simulink model "TRAMI_STEP_AT_vehicle_ver01_R2018b"  (R2018b)
settings: Solver=ode8  StartTime=0  StopTime=end_time  FixedStep=sampling_time  RelTol=1e-3
StartFcn:
  | csvwrite('simstart.csv',1)
StopFcn:
  | csvwrite('simstop.csv',1)
values from neighbouring files (symbols this model uses):
  sampling_time = 0.0025    [METI_TRAMI_Thermal_ver01_Jmaab_PreLoad.m]
undefined symbols (not defined in the file or in its folder): ACC_D_Gain, ACC_I_Gain, ACC_P_Gain, ALT_CNT_ALT_OFF_RPM_HYS_rpm, ALT_CNT_ALT_ON_RPM_HYS_rpm, ALT_CNT_Alter_V_BASE_V, ALT_CNT_Alter_V_Kaisei_V, ALT_CNT_flag_disable_kaisei, ALT_CNT_V_Battely_Kudo_V, ALT_PNT_ALT_GDCurrent_A, ALT_PNT_ALT_GDVolt_V, ALT_PNT_Alter_limit_Current_V_table, ALT_PNT_Alter_limit_Current_V_table_x_rpm, ALT_PNT_Alter_trq_Nm_map, ALT_PNT_Alter_trq_Nm_map_x_rpm, ALT_PNT_Alter_trq_Nm_map_y_Current_A, ALT_PNT_Alter_trq_Nm_map_z_Volt_tgt_V, ALT_PNT_eta_pulley_alt, ALT_PNT_Gain_Alt_v_del, ALT_PNT_ratio_pulley_alt, ALT_PNT_Tau_Alternator_V_tgt_s, ALT_PNT_trq_alter_output_LL_Nm, BK_PNT_Pow_UL, BK_PNT_Tau_brake, Brk_LL, Brk_PGain, Brk_UL, BT_PNT_Lo_Capa_lo_batt_F, BT_PNT_Lo_ocv_SOC_lo_batt_OCV_V_table, BT_PNT_Lo_ocv_SOC_lo_batt_OCV_V_table_x_SOC, BT_PNT_Lo_R_lo_batt_ohm, BT_PNT_Lo_SOC_MAX_lo_batt, BT_PNT_Lo_SOC_MIN_lo_batt, BT_PNT_Lo_SOC_START_lo_batt, BT_PNT_Lo_V_start_ocv, Driver_Brake_Const1, Driver_Brake_Const3, Driver_Brake_Switch_Const2, Driver_Brk_sh, drivmode_ACC, drivmode_CONST, drivmode_GensokuKaisei, drivmode_GensokuRikko, drivmode_STOP, EL_PNT_R_bodyelec_lo_ohm, ENG_CNT_Accel_LL, ENG_CNT_Accel_UL, ENG_CNT_brak_idlestop, ENG_CNT_flag_idle_stop_exe, ENG_CNT_gain_p_per_isc, ENG_CNT_IdleSpeed_Const, ENG_CNT_omg_eng_fuelcut_rpm, ENG_CNT_per_isc_max, ENG_CNT_per_isc_min, ENG_CNT_per_throttle_fuelcut, ENG_CNT_per_throttle_isc_fb, ENG_CNT_Starter_timer_Const_s, ENG_CNT_Throttle_LL, ENG_CNT_Throttle_UL, ENG_CNT_V_car_idlestop_kmph ... (+29)
libraries: METI_Lib_vehicle_model x18, simulink x4, AZAPA_Lib_vehicle_model x1
(part 1 of 2)
settings Model: SimulationMode=accelerator  Creator=nishimura  LastModifiedBy=kotaroy
settings SolverCC: AlgebraicLoopSolver=LineSearch
settings DataIOCC: SaveFormat=Array  SaveOutput=off  SignalLogging=off  DSMLogging=off  SaveTime=off
settings OptimizationCC: BlockReduction=off  BooleanDataType=off  EfficientMapNaN2IntZero=off  LifeSpan=inf
settings DebuggingCC: SaveWithParameterizedLinksMsg=none  UnderspecifiedInitializationDetection=Classic  MergeDetectMultiDrivingBlocksExec=none  SignalResolutionControl=TryResolveAllWithWarning  ParameterPrecisionLossMsg=none  AllowSymbolicDim=off  StrictBusMsg=ErrorOnBusTreatedAsVector  SFUnexpectedBacktrackingDiag=warning  SFNoUnconditionalDefaultTransitionDiag=warning  SFExecutionAtInitializationDiag=none
settings HardwareCC: ProdBitPerPointer=32  ProdBitPerSizeT=32  ProdBitPerPtrDiffT=32  ProdLargestAtomicFloat=None  ProdIntDivRoundTo=Undefined  ProdEndianess=Unspecified  ProdWordSize=32  ProdHWDeviceType=32-bit Generic  TargetBitPerPointer=64  TargetBitPerSizeT=64  TargetBitPerPtrDiffT=64  TargetLongLongMode=on  TargetIntDivRoundTo=Zero  TargetEndianess=LittleEndian  TargetWordSize=64  TargetHWDeviceType=MATLAB Host  ProdEqTarget=off
settings ModelReferenceCC: PropagateSignalLabelsOutOfModel=off
settings SFSimCC: SimUseLocalCustomCode=off
settings CodeAppCC: MaxIdLength=128
settings GRTTargetCC: TargetLangStandard=C89/C90 (ANSI)  CombineOutputUpdateFcns=off  GRTInterface=on
settings ConfigComp: CovMetricSettings=dw  CovHtmlReporting=on  CovSaveCumulativeToWorkspaceVar=on  CovSaveSingleToWorkspaceVar=on  CovExternalEMLEnable=off  CovSFcnEnable=off

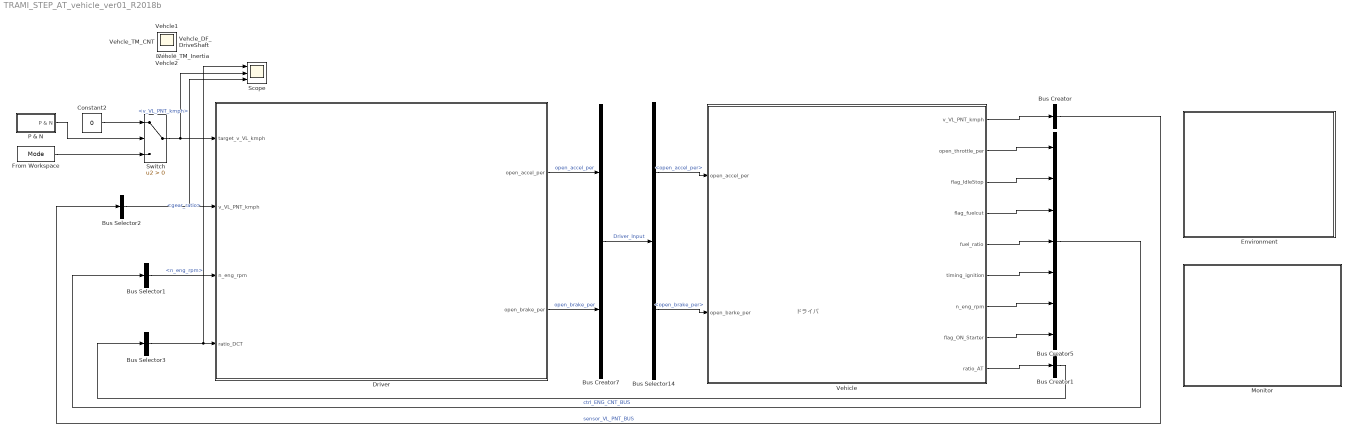
== system TRAMI_STEP_AT_vehicle_ver01_R2018b ==
  note: ドライバ
  Bus Creator : BusCreator  Inputs=1
  Bus Creator1 : BusCreator  Inputs=1
  Bus Creator5 : BusCreator  Inputs=7
  Bus Creator7 : BusCreator  Inputs=2
  Bus Selector1 : BusSelector  OutputSignals=n_eng_rpm
  Bus Selector14 : BusSelector  OutputSignals=open_accel_per,open_brake_per
  Bus Selector2 : BusSelector  OutputSignals=v_VL_PNT_kmph
  Bus Selector3 : BusSelector  OutputSignals=gear_ratio
  Constant2 : Constant  Value=0
  Driver : Subsystem
      mask Display: image(imread('picture\ドライバ.png'))
  Environment : Subsystem
      mask Display: image(imread('picture\外部環境.png'))
  From Workspace : FromWorkspace  VariableName=Mode  SampleTime=0  OutputAfterFinalValue=Holding final value
  Monitor : Subsystem
  P & N : Subsystem
  Scope : Scope  NumInputPorts=3
  Switch : Switch  Criteria=u2 > Threshold
  Vehicle : Subsystem
      mask Display: image(imread('picture\電気負荷.png'))
  Driver1 : Scope
  Vehcle1 : Scope
  Vehcle2 : Scope
  Vehcle_DF_DriveShaft : Scope
  Vehcle_TM_CNT : Scope
  Vehcle_TM_Inertia : Scope
  wires:
  Bus Creator7/1 -> Bus Selector14/1  "Driver_Input"
  Bus Creator/1 -> Bus Selector2/1  "sensor_VL_PNT_BUS"
  Bus Creator5/1 -> Bus Selector1/1  "ctrl_ENG_CNT_BUS"
  Vehicle/1(v_VL_PNT_kmph) -> Bus Creator/1
  Vehicle/2(open_throttle_per) -> Bus Creator5/1
  Vehicle/3(flag_IdleStop) -> Bus Creator5/2
  Vehicle/4(flag_fuelcut) -> Bus Creator5/3
  Vehicle/5(fuel_ratio) -> Bus Creator5/4
  Vehicle/6(timing_ignition) -> Bus Creator5/5
  Vehicle/7(n_eng_rpm) -> Bus Creator5/6
  Vehicle/8(flag_ON_Starter) -> Bus Creator5/7
  Bus Selector14/1 -> Vehicle/1(open_accel_per)  "<open_accel_per>"
  Bus Selector14/2 -> Vehicle/2(open_barke_per)  "<open_brake_per>"
  Driver/1(open_accel_per) -> Bus Creator7/1  "open_accel_per"
  Driver/2(open_brake_per) -> Bus Creator7/2  "open_brake_per"
  Bus Selector1/1 -> Driver/3(n_eng_rpm)  "<n_eng_rpm>"
  Switch/1 -> Scope/2, Driver/1(target_v_VL_kmph)
  Constant2/1 -> Switch/1
  P & N/1(P & N) -> Switch/2
  From Workspace/1 -> Switch/3
  Vehicle/9(ratio_AT) -> Bus Creator1/1
  Bus Creator1/1 -> Bus Selector3/1
  Bus Selector3/1 -> Scope/1, Driver/4(ratio_DCT)  "<gear_ratio>"
  Bus Selector2/1 -> Scope/3, Driver/2(v_VL_PNT_kmph)  "<v_VL_PNT_kmph>"

== system TRAMI_STEP_AT_vehicle_ver01_R2018b/Driver ==
  note: ドライバモデルのへたくそ対応
  note: 全体としてパワーを算出しておいて、
      | さらにパワーと速度のF/Bを切り替えれるようにしておく
  target_v_VL_kmph : Inport
  v_VL_PNT_kmph : Inport  Port=2
  n_eng_rpm : Inport  Port=3
  ratio_DCT : Inport  Port=4
  Caliculate_Driving_State : Subsystem
  Caliculate_Opeining_Accel : Subsystem
  Caliculate_Opening_Brake : Subsystem
  Memory2 : Memory  InheritSampleTime=on
  Memory3 : Memory
  Memory4 : Memory
  open_accel_per : Outport
  open_brake_per : Outport  Port=2
  tag scope: tScope_accel=global, tScope_brake=global
  wires:
  target_v_VL_kmph/1 -> Caliculate_Opeining_Accel/2(target_v_VL_kmph), Caliculate_Opening_Brake/2(target_v_VL_kmph), Caliculate_Driving_State/2(target_v_VL_kmph)
  Memory3/1 -> Caliculate_Opeining_Accel/3(pre_n_eng_rpm)  "pre_n_eng_rpm"
  Memory4/1 -> Caliculate_Opeining_Accel/4(pre_ratio_DCT)
  n_eng_rpm/1 -> Memory3/1
  Memory2/1 -> Caliculate_Opening_Brake/1(v_VL_PNT_kmph), Caliculate_Opeining_Accel/1(v_VL_PNT_kmph)
  Caliculate_Opening_Brake/1(open_brake_per) -> open_brake_per/1, [tScope_brake], Caliculate_Driving_State/1(open_brake_per)
  v_VL_PNT_kmph/1 -> Memory2/1
  ratio_DCT/1 -> Memory4/1
  Caliculate_Opeining_Accel/1(open_accel_per) -> [tScope_accel], open_accel_per/1, Caliculate_Opening_Brake/3(open_accel_per)

== system TRAMI_STEP_AT_vehicle_ver01_R2018b/Environment ==
  note: 登坂。風、温度、湿度・・・
  Clock : Clock
  To Workspace : ToWorkspace  VariableName=simtime  SampleTime=-1
      settings: Decimation=num_tws_mabiki
  wires:
  Clock/1 -> To Workspace/1

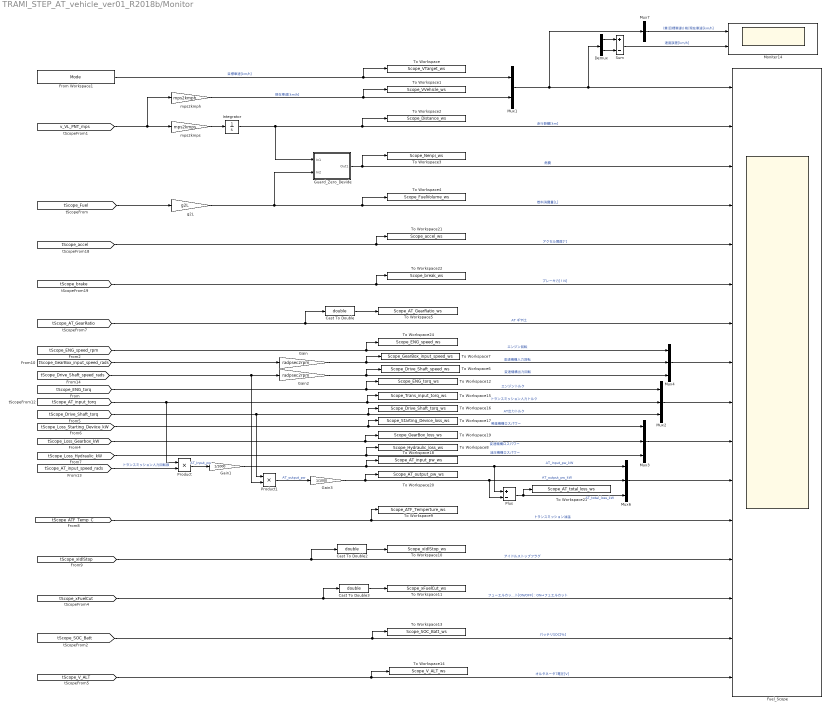
== system TRAMI_STEP_AT_vehicle_ver01_R2018b/Monitor ==
  Cast To Double : DataTypeConversion  OutDataTypeStr=double
  Cast To Double2 : DataTypeConversion  OutDataTypeStr=double
  Cast To Double3 : DataTypeConversion  OutDataTypeStr=double
  Demux : Demux  Outputs=2
  From Workspace1 : FromWorkspace  VariableName=Mode  SampleTime=0  OutputAfterFinalValue=Holding final value
  Fuel_Scope : Scope  NumInputPorts=16
  Gain : Gain  Tag=単位変換  Gain=radpsec2rpm
  Gain1 : Gain  Gain=1/1000
  Gain2 : Gain  Tag=単位変換  Gain=radpsec2rpm
  Gain3 : Gain  Gain=1/1000
  Guard_Zero_Devide : Subsystem
  Integrator : Integrator
  Moniter14 : Scope  NumInputPorts=2
  Mux1 : Mux  Inputs=2
  Mux{2..4,6} (4 alike) : Mux  Inputs=3
  Mux7 : Mux  Inputs=1
  Plus : Sum  Inputs=+-
  Product : Product
  Product1 : Product
  Sum : Sum  Inputs=+-
  To Workspace : ToWorkspace  VariableName=Scope_VTarget_ws  SampleTime=-1
      settings: Decimation=num_tws_mabiki
  To Workspace1 : ToWorkspace  VariableName=Scope_VVehicle_ws  SampleTime=-1
      settings: Decimation=num_tws_mabiki
  To Workspace10 : ToWorkspace  VariableName=Scope_xIdlStop_ws  SampleTime=-1
      settings: Decimation=num_tws_mabiki
  To Workspace11 : ToWorkspace  VariableName=Scope_xFuelCut_ws  SampleTime=-1
      settings: Decimation=num_tws_mabiki
  To Workspace12 : ToWorkspace  VariableName=Scope_ENG_torq_ws  SampleTime=-1
      settings: Decimation=num_tws_mabiki
  To Workspace13 : ToWorkspace  VariableName=Scope_SOC_Batt_ws  SampleTime=-1
      settings: Decimation=num_tws_mabiki
  To Workspace14 : ToWorkspace  VariableName=Scope_V_ALT_ws  SampleTime=-1
      settings: Decimation=num_tws_mabiki
  To Workspace15 : ToWorkspace  VariableName=Scope_Trans_input_torq_ws  SampleTime=-1
      settings: Decimation=num_tws_mabiki
  To Workspace16 : ToWorkspace  VariableName=Scope_Drive_Shaft_torq_ws  SampleTime=-1
      settings: Decimation=num_tws_mabiki
  To Workspace17 : ToWorkspace  VariableName=Scope_Starting_Device_loss_ws  SampleTime=-1
      settings: Decimation=num_tws_mabiki
  To Workspace18 : ToWorkspace  VariableName=Scope_AT_input_pw_ws  SampleTime=-1
      settings: Decimation=num_tws_mabiki
  To Workspace19 : ToWorkspace  VariableName=Scope_GearBox_loss_ws  SampleTime=-1
      settings: Decimation=num_tws_mabiki
  To Workspace2 : ToWorkspace  VariableName=Scope_Distance_ws  SampleTime=-1
      settings: Decimation=num_tws_mabiki
  To Workspace20 : ToWorkspace  VariableName=Scope_AT_output_pw_ws  SampleTime=-1
      settings: Decimation=num_tws_mabiki
  To Workspace21 : ToWorkspace  VariableName=Scope_accel_ws  SampleTime=-1
      settings: Decimation=num_tws_mabiki
  To Workspace22 : ToWorkspace  VariableName=Scope_break_ws  SampleTime=-1
      settings: Decimation=num_tws_mabiki
  To Workspace24 : ToWorkspace  VariableName=Scope_ENG_speed_ws  SampleTime=-1
      settings: Decimation=num_tws_mabiki
  To Workspace25 : ToWorkspace  VariableName=Scope_AT_total_loss_ws  SampleTime=-1
      settings: Decimation=num_tws_mabiki
  To Workspace3 : ToWorkspace  VariableName=Scope_Nenpi_ws  SampleTime=-1
      settings: Decimation=num_tws_mabiki
  To Workspace4 : ToWorkspace  VariableName=Scope_FuelVolume_ws  SampleTime=-1
      settings: Decimation=num_tws_mabiki
  To Workspace5 : ToWorkspace  VariableName=Scope_AT_GearRatio_ws  SampleTime=-1
      settings: Decimation=num_tws_mabiki
  To Workspace6 : ToWorkspace  VariableName=Scope_Drive_Shaft_speed_ws  SampleTime=-1
      settings: Decimation=num_tws_mabiki
  To Workspace7 : ToWorkspace  VariableName=Scope_GearBox_input_speed_ws  SampleTime=-1
      settings: Decimation=num_tws_mabiki
  To Workspace8 : ToWorkspace  VariableName=Scope_Hydraulic_loss_ws  SampleTime=-1
      settings: Decimation=num_tws_mabiki
  To Workspace9 : ToWorkspace  VariableName=Scope_ATF_Temperture_ws  SampleTime=-1
      settings: Decimation=num_tws_mabiki
  g2L : Gain  Gain=g2L
  mps2kmph : Gain  Gain=mps2kmph
  mps2kmps : Gain  Gain=mps2kmps
  wires:
  [tScope_xFuelCut] -> Fuel_Scope/14, Cast To Double3/1  "フューエルカット[ON/OFF] : ON→フュエルカット"
  [v_VL_PNT_mps] -> mps2kmph/1, mps2kmps/1
  mps2kmps/1 -> Integrator/1
  [tScope_Fuel] -> g2L/1
  Integrator/1 -> Guard_Zero_Devide/1(In1), Fuel_Scope/2, To Workspace2/1  "走行距離[km]"
  g2L/1 -> Fuel_Scope/4, To Workspace4/1, Guard_Zero_Devide/2(In2)  "燃料消費量[L]"
  [tScope_ATF_Temp_C] -> Fuel_Scope/12, To Workspace9/1  "トランスミッション油温"
  From Workspace1/1 -> To Workspace/1, Mux1/1  "目標車速[km/h]"
  mps2kmph/1 -> To Workspace1/1, Mux1/2  "現在車速[km/h]"
  Mux1/1 -> Mux7/1, Fuel_Scope/1, Demux/1
  [tScope_Loss_Gearbox_kW] -> To Workspace19/1, Mux3/2  "変速機構ロスパワー"
  [tScope_Drive_Shaft_torq] -> Product1/1, To Workspace16/1, Mux2/3  "AT出力トルク"
  Mux3/1 -> Fuel_Scope/10
  [tScope_accel] -> Fuel_Scope/5, To Workspace21/1  "アクセル開度[°]"
  [tScope_brake] -> Fuel_Scope/6, To Workspace22/1  "ブレーキ力[１N]"
  [tScope_ENG_speed_rpm] -> To Workspace24/1, Mux4/1  "エンジン回転"
  Demux/1 -> Sum/1
  Demux/2 -> Sum/2
  Sum/1 -> Moniter14/2  "速度誤差[km/h]"
  [tScope_V_ALT] -> Fuel_Scope/16, To Workspace14/1  "オルタネータ7電圧[V]"
  [tScope_SOC_Batt] -> Fuel_Scope/15, To Workspace13/1  "バッテリSOC[%]"
  Guard_Zero_Devide/1(Out1) -> Fuel_Scope/3, To Workspace3/1  "燃費"
  Gain/1 -> Mux4/2, To Workspace7/1  "変速機構入力回転"
  [tScope_ENG_torq] -> To Workspace12/1, Mux2/1  "エンジントルク"
  [tScope_AT_input_torq] -> Mux2/2, To Workspace15/1, Product/1  "トランスミッション入力トルク"
  [tScope_Loss_Starting_Deviice_kW] -> To Workspace17/1, Mux3/1  "発進機構ロスパワー"
  [tScope_Loss_Hydraulic_kW] -> To Workspace8/1, Mux3/3  "油圧機構ロスパワー"
  Mux2/1 -> Fuel_Scope/9
  [tScope_xIdlStop] -> Fuel_Scope/13, Cast To Double2/1  "アイドルストップフラグ"
  Mux4/1 -> Fuel_Scope/8
  Cast To Double3/1 -> To Workspace11/1
  Cast To Double2/1 -> To Workspace10/1
  [tScope_GearBox_input_speed_rads] -> Gain/1
  Gain2/1 -> To Workspace6/1, Mux4/3  "変速機構出力回転"
  [tScope_Drive_Shaft_speed_rads] -> Product1/2, Gain2/1
  Mux6/1 -> Fuel_Scope/11
  Gain1/1 -> To Workspace18/1, Mux6/1, Plus/1  "AT_Input_pw_kW"
  [tScope_AT_input_speed_rads] -> Product/2  "トランスミッション入力回転数"
  Product1/1 -> Gain3/1  "AT_output_pw"
  Plus/1 -> To Workspace25/1, Mux6/3  "AT_total_loss_kW"
  Product/1 -> Gain1/1  "AT_Input_pw"
  Gain3/1 -> To Workspace20/1, Plus/2, Mux6/2  "AT_output_pw_kW"
  Cast To Double/1 -> To Workspace5/1
  [tScope_AT_GearRatio] -> Cast To Double/1, Fuel_Scope/7  "AT ギヤ比"
  Mux7/1 -> Moniter14/1  "(黄)目標車速/(桃)現在車速[km/h]"

== system TRAMI_STEP_AT_vehicle_ver01_R2018b/P & N ==
  Constant : Constant
  Constant1 : Constant  Value=3
  Logical Operator : Logic  Operator=OR  AllPortsSameDT=off  OutDataTypeStr=boolean
  Relational Operator : RelationalOperator  Operator===  OutDataTypeStr=boolean  RndMeth=Simplest
  Relational Operator1 : RelationalOperator  Operator===  OutDataTypeStr=boolean  RndMeth=Simplest
  shift_range : Constant  Value=4
  P & N : Outport
  wires:
  shift_range/1 -> Relational Operator/1, Relational Operator1/1
  Relational Operator1/1 -> Logical Operator/1
  Logical Operator/1 -> P & N/1
  Relational Operator/1 -> Logical Operator/2
  Constant/1 -> Relational Operator/2
  Constant1/1 -> Relational Operator1/2

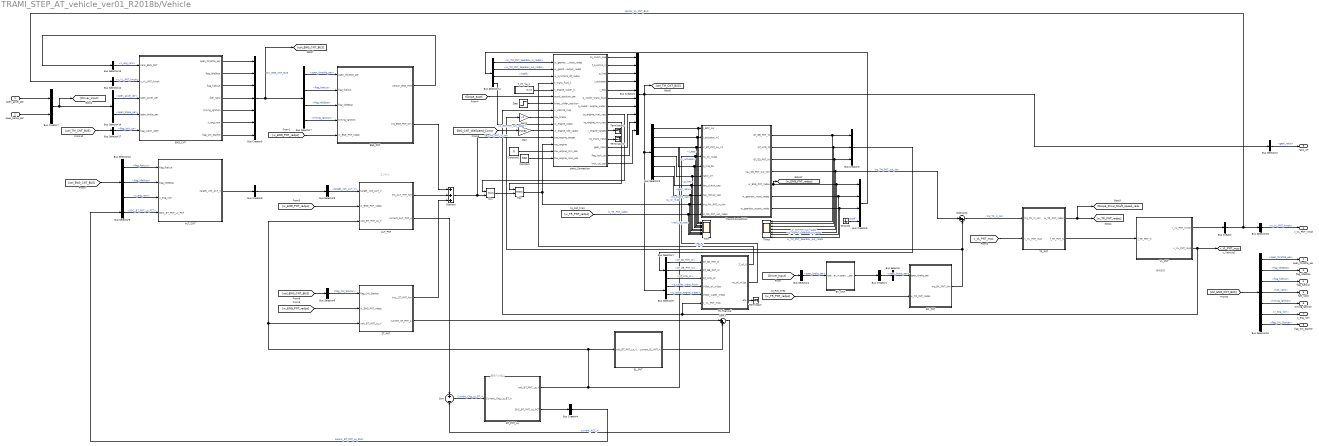
== system TRAMI_STEP_AT_vehicle_ver01_R2018b/Vehicle ==
  note: エンジン
  note: 低圧バッテリ
  note: 車両抵抗
  open_accel_per : Inport
  open_barke_per : Inport  Port=2
  ALT_CNT : Subsystem
      mask Display: image(imread('picture\ECU.png'))
  ALT_PNT : Subsystem
      mask Display: image(imread('picture\image\オルタネータ02.jpg'))
  BK_CNT : Subsystem
      mask Display: image(imread('picture\ECU.png'))
  BK_PNT : Subsystem
      mask Display: image(imread('picture\ブレーキ02.png'))
  BT_PNT_Lo : Subsystem
      mask Display: image(imread('picture\バッテリー.png'))
  Bus Creator{,1,4,6} (4 alike) : BusCreator  Inputs=1
  Bus Creator2 : BusCreator  Inputs=10
  Bus Creator3 : BusCreator  Inputs=3
  Bus Creator5 : BusCreator  Inputs=7
  Bus Creator7 : BusCreator  Inputs=2
  Bus Creator8 : BusCreator  Inputs=4
  Bus Selector : BusSelector  OutputSignals=open_brake_per
  Bus Selector1 : BusSelector  OutputSignals=Qf_SD_PNT_W,Qf_GB_PNT_W,Qf_HYD_W
  Bus Selector10 : BusSelector  OutputSignals=flag_fuelcut,flag_IdleStop,n_eng_rpm
  Bus Selector11 : BusSelector  OutputSignals=w_TM_PNT_GearBox_in_radps,w_TM_PNT_GearBox_out_radps,wDiff,w_TM_PNT_out_radps
  Bus Selector12 : BusSelector  OutputSignals=v_VL_PNT_kmph
  Bus Selector13 : BusSelector  OutputSignals=n_eng_rpm
  Bus Selector14 : BusSelector  OutputSignals=open_accel_per,open_brake_per
  Bus Selector15 : BusSelector  OutputSignals=open_throttle_per,flag_IdleStop,flag_fuelcut,fuel_ratio,timing_ignition,n_eng_rpm,flag_ON_Starter
  Bus Selector16 : BusSelector  OutputSignals=v_VL_PNT_kmph
  Bus Selector17 : BusSelector  OutputSignals=flag_lock_up
  Bus Selector2 : BusSelector  OutputSignals=gear_ratio
  Bus Selector3 : BusSelector  OutputSignals=i_eop,i_actuator,p_line,gear_ratio,tq_clutch_cap,lock_up_cap
  Bus Selector4 : BusSelector  OutputSignals=open_brake_per
  Bus Selector5 : BusSelector  OutputSignals=q_cooler_trans_fluid,q_cooler_engine_water
  Bus Selector6 : BusSelector  OutputSignals=flag_ON_Starter
  Bus Selector7 : BusSelector  OutputSignals=open_throttle_per,flag_fuelcut,flag_IdleStop,timing_ignition
  Bus Selector8 : BusSelector  OutputSignals=target_volt_ALT_V
  Bus Selector9 : BusSelector  OutputSignals=SOC_BT_PNT_Lo_PCT
  Constant : Constant  Value=500
  Constant1 : Constant  Value=0
  EL_PNT : Subsystem
      mask Display: image(imread('picture\電気負荷.png'))
  ENG_CNT : Subsystem
      mask Display: image(imread('picture\ECU.png'))
  ENG_PNT : Subsystem
      mask Display: image(imread('picture\image\エンジン03.jpg'))
  Gain : Gain  Gain=2*pi/60
  Gain1 : Gain  Gain=-1
  Ground1 : Ground
  Max : MinMax  Function=max  Inputs=2
  Min : MinMax  Inputs=2
  ST_PNT : Subsystem
      mask Display: image(imread('picture\image\スターター02.jpg'))
  Step : Step  Time=5.57  SampleTime=0
  Subtract : Sum  Inputs=3
  Subtract2 : Sum  Inputs=|++
  Sum : Sum  Inputs=+|-
  Sum1 : Sum  Inputs=|++
  TM Thermal : Subsystem
  TMin : Scope  NumInputPorts=10
  TMout : Scope  NumInputPorts=7
  TR_PNT : Subsystem
      mask Display: image(imread('picture\タイヤ01.png'))
  T_PT_TH_K : Subsystem
  Terminator : Terminator
  Terminator1 : Terminator
  Terminator2 : Terminator
  TransmissionFMU2 : Subsystem
  VL_PNT : Subsystem
      mask Display: image(imread('picture\車両抵抗.png'))
  plant_Connection : Subsystem
  v_VL_PNT_kmph : Outport
  open_throttle_per : Outport  Port=2
  flag_IdleStop : Outport  Port=3
  flag_fuelcut : Outport  Port=4
  fuel_ratio : Outport  Port=5
  timing_ignition : Outport  Port=6
  n_eng_rpm : Outport  Port=7
  flag_ON_Starter : Outport  Port=8
  ratio_AT : Outport  Port=9
  tag scope: tScope_Drive_Shaft_speed_rads=global, v_VL_PNT_mps=global
  wires:
  Bus Creator7/1 -> Bus Selector14/1, [Driver_Input]
  ENG_PNT/1(sensor_ENG_PNT) -> Bus Selector13/1
  Sum/1 -> BT_PNT_Lo/1(Current_Chg_Lo_BT_A)  "Current_Chg_Lo_BT_A"
  EL_PNT/1(current_EL_PNT_A) -> Sum1/2
  ALT_PNT/2(current_ALT_PNT_A) -> Sum/1
  Bus Creator5/1 -> Bus Selector7/1, [ctrl_ENG_CNT_BUS]  "ctrl_ENG_CNT_BUS"
  Bus Creator6/1 -> Bus Selector8/1
  ST_PNT/2(current_ST_PNT_A) -> Sum1/1
  BT_PNT_Lo/1(volt_BT_PNT_Lo_V) -> TransmissionFMU2/3(V_BT_PNT_Lo_V1), TMin/3, EL_PNT/1(volt_BT_PNT_Lo_V), ST_PNT/3(volt_BT_PNT_Lo_V), ALT_PNT/3(volt_BT_PNT_Lo_V)
  Subtract/1 -> plant_Connection/12(tau_engine_target), Min/2  "tau_FW_PNT_in_Nm"
  ENG_PNT/2(trq_ENG_PNT_Nm) -> Subtract/1
  ST_PNT/1(trq__ST_PNT_Nm) -> Subtract/3
  [w_ENG_PNT_radps] -> ALT_PNT/2(w_ENG_PNT_radps)
  [ctrl_ENG_CNT_BUS] -> Bus Selector10/1
  [ctrl_ENG_CNT_BUS] -> Bus Selector6/1
  Sum1/1 -> Sum/2  "current_ACC_A"
  [w_ENG_PNT_radps] -> ST_PNT/2(w_ENG_PNT_radps)
  Bus Creator/1 -> Bus Selector16/1, Bus Selector12/1  "sensor_VL_PNT_BUS"
  TR_PNT/2(f_TR_PNT_N) -> VL_PNT/1(f_TR_PNT_N)
  Subtract2/1 -> TR_PNT/1(trq_TR_in_Nm)  "trq_TR_in_Nm"
  [w_TR_PNT_radps] -> BK_PNT/2(w_TR_PNT_radps)
  [v_VL_PNT_mps] -> TR_PNT/2(v_VL_PNT_mps)
  [Driver_Input] -> Bus Selector4/1
  VL_PNT/1(v_VL_PNT_kmph) -> Bus Creator/1
  Bus Creator1/1 -> Bus Selector/1
  BK_CNT/1(open_brake_per) -> Bus Creator1/1
  Bus Selector/1 -> BK_PNT/1(open_brake_per)  "<open_brake_per>"
  Bus Selector4/1 -> BK_CNT/1(open_brake_per_in)  "<open_brake_per>"
  Bus Creator4/1 -> Bus Selector9/1  "sensor_BT_PNT_Lo_BUS"
  BT_PNT_Lo/2(SOC_BT_PNT_Lo_PCT) -> Bus Creator4/1
  Bus Selector6/1 -> ST_PNT/1(flag_ON_Starter)  "<flag_ON_Starter>"
  Bus Selector7/1 -> ENG_PNT/1(open_throttle_per)  "<open_throttle_per>"
  Bus Selector7/2 -> ENG_PNT/2(flag_fuelcut)  "<flag_fuelcut>"
  Bus Selector7/3 -> ENG_PNT/3(flag_IdleStop)  "<flag_IdleStop>"
  Bus Selector7/4 -> ENG_PNT/4(timing_ignition)  "<timing_ignition>"
  ENG_CNT/1(open_throttle_per) -> Bus Creator5/1
  ENG_CNT/7(flag_ON_Starter) -> Bus Creator5/7
  ENG_CNT/6(n_eng_rpm) -> Bus Creator5/6
  ENG_CNT/5(timing_ignition) -> Bus Creator5/5
  ENG_CNT/4(fuel_ratio) -> Bus Creator5/4
  ENG_CNT/3(flag_fuelcut) -> Bus Creator5/3
  ENG_CNT/2(flag_IdleStop) -> Bus Creator5/2
  Bus Selector8/1 -> ALT_PNT/1(target_volt_ALT_V)  "<target_volt_ALT_V>"
  ALT_CNT/1(target_volt_ALT_V) -> Bus Creator6/1
  Bus Selector9/1 -> ALT_CNT/4(SOC_BT_PNT_Lo_PCT)  "<SOC_BT_PNT_Lo_PCT>"
  Bus Selector10/1 -> ALT_CNT/1(flag_fuelcut)  "<flag_fuelcut>"
  Bus Selector10/2 -> ALT_CNT/2(flag_IdleStop)  "<flag_IdleStop>"
  Bus Selector10/3 -> ALT_CNT/3(n_eng_rpm)  "<n_eng_rpm>"
  Bus Selector12/1 -> ENG_CNT/2(v_VL_PNT_kmph)  "<v_VL_PNT_kmph>"
  Bus Selector13/1 -> ENG_CNT/1(sens_ENG_PNT)  "<n_eng_rpm>"
  Bus Selector14/1 -> ENG_CNT/3(open_accel_per)  "<open_accel_per>"
  [ctrl_ENG_CNT_BUS] -> Bus Selector15/1
  Bus Selector16/1 -> v_VL_PNT_kmph/1  "<v_VL_PNT_kmph>"
  Bus Selector15/1 -> open_throttle_per/1  "<open_throttle_per>"
  Bus Selector15/3 -> flag_fuelcut/1  "<flag_fuelcut>"
  Bus Selector15/2 -> flag_IdleStop/1  "<flag_IdleStop>"
  Bus Selector15/4 -> fuel_ratio/1  "<fuel_ratio>"
  Bus Selector15/5 -> timing_ignition/1  "<timing_ignition>"
  Bus Selector15/6 -> n_eng_rpm/1  "<n_eng_rpm>"
  Bus Selector15/7 -> flag_ON_Starter/1  "<flag_ON_Starter>"
  open_accel_per/1 -> Bus Creator7/1
  open_barke_per/1 -> Bus Creator7/2
  BK_PNT/1(trq_BK_PNT_Nm) -> Gain1/1, Subtract2/2
  VL_PNT/2(v_VL_PNT_mps) -> plant_Connection/8(v_vehicle_mps), TM Thermal/6(v_VL_PNT_mps), [v_VL_PNT_mps]
  TM Thermal/3(eta) -> Terminator/1
  Bus Creator2/1 -> Bus Selector2/1, [ctrl_TM_CNT_BUS], Bus Selector5/1, Bus Selector3/1
  Bus Selector3/5 -> TransmissionFMU2/7(tau_clutch_cap), TMin/7  "<tq_clutch_cap>"
  Bus Creator3/1 -> Bus Selector1/1
  [tScope_accel] -> plant_Connection/6(accel_position_per)
  Bus Selector5/1 -> TM Thermal/4(VlDot_oil_m3ps)  "<q_cooler_trans_fluid>"
  Bus Selector5/2 -> TM Thermal/5(VlDot_water_m3ps)  "<q_cooler_engine_water>"
  TM Thermal/1(T_oil_K) -> plant_Connection/4(t_trans_fluid_k)  "T_oil_K"
  [w_ENG_PNT_radps] -> ENG_PNT/5(w_ENG_PNT_radps)
  [ctrl_TM_CNT_BUS] -> Bus Selector17/1
  Bus Selector14/2 -> ENG_CNT/4(open_brake_per)  "<open_brake_per>"
  Bus Selector17/1 -> ENG_CNT/5(flag_cutch_open)  "<flag_lock_up>"
  TR_PNT/1(w_TR_PNT_radps) -> [tScope_Drive_Shaft_speed_rads], [w_TR_PNT_radps]
  TransmissionFMU2/4(tau_DS_PNT_out_Nm) -> TMout/4, Subtract2/1  "trq_TM_PNT_out_Nm"
  Ground1/1 -> Bus Creator8/4  "wDiff"
  Bus Selector11/4 -> plant_Connection/10(w_engine_radps)  "<w_TM_PNT_out_radps>"
  Bus Selector11/3 -> plant_Connection/3(w_synchoro_dif_radps)  "<wDiff>"
  ALT_PNT/1(trq_ALT_PNT_Nm) -> Subtract/2
  Min/1 -> Max/2
  plant_Connection/9(tq_engine_min_req) -> Max/1
  plant_Connection/8(tq_engine_max_req) -> Min/1
  TransmissionFMU2/6(w_gearbox_input_radps) -> TMout/6, Bus Creator8/2  "w_TM_PNT_GearBox_in_radps"
  Step/1 -> plant_Connection/7(trans_shifer_position)
  [ENG_CNT_IdleSpeed_Const] -> Gain/1
  Constant1/1 -> plant_Connection/14(tau_engine_min_pos)
  Constant/1 -> plant_Connection/15(tau_engine_max_pos)
  TransmissionFMU2/1(Qf_GB_PNT_W) -> TMout/1, Bus Creator3/1
  TransmissionFMU2/7(w_gearbox_output_radps) -> TMout/7, Bus Creator8/3  "w_TM_PNT_GearBox_out_radps"
  TransmissionFMU2/5(w_ENG_PNT_radps) -> [w_ENG_PNT_radps], TMout/5, Bus Creator8/1  "w_TM_PNT_out_radps"
  Bus Selector11/1 -> plant_Connection/1(w_gearbox_input_radps)  "<w_TM_PNT_GearBox_in_radps>"
  Bus Selector11/2 -> plant_Connection/2(w_gearbox_output_radps)  "<w_TM_PNT_GearBox_out_radps>"
  plant_Connection/1(tq_clutch_cap) -> Bus Creator2/1
  plant_Connection/2(f_synchro_n) -> Bus Creator2/2
  plant_Connection/3(p_line) -> Bus Creator2/3
  plant_Connection/4(i_actuator) -> Bus Creator2/4
  plant_Connection/5(i_eop) -> Bus Creator2/5
  plant_Connection/6(q_cooler_trans_fluid) -> Bus Creator2/6
  plant_Connection/7(q_cooler_engine_water) -> Bus Creator2/7
  plant_Connection/10(r_engine_target) -> Terminator1/1
  plant_Connection/11(tq_trans_input) -> Terminator2/1
  plant_Connection/12(gear_ratio) -> Bus Creator2/8
  Bus Selector3/3 -> TransmissionFMU2/5(p_line_Pa), TMin/5  "<p_line>"
  Max/1 -> TransmissionFMU2/9(trq_FW_PNT_in_Nm), TMin/9, plant_Connection/13(tau_engine)
  [w_TR_PNT_radps] -> TransmissionFMU2/10(w_DS_PNT_out_radps), TMin/10  "w_TR_PNT_radps"
  Gain/1 -> plant_Connection/11(w_engine_idle_radps)
  Gain1/1 -> plant_Connection/9(tau_brake)
  Bus Selector1/1 -> TM Thermal/1(Qf_SD_PNT_W)  "<Qf_SD_PNT_W>"
  Bus Selector1/3 -> TM Thermal/3(Qf_HYD_W)  "<Qf_HYD_W>"
  Bus Selector1/2 -> TM Thermal/2(Qf_GB_PNT_W)  "<Qf_GB_PNT_W>"
  Bus Selector3/4 -> TransmissionFMU2/6(ratio_AT), TMin/6  "<gear_ratio>"
  Bus Selector3/6 -> TransmissionFMU2/8(tau_lockup_cap), TMin/8  "<lock_up_cap>"
  plant_Connection/13(flag_lock_up) -> Bus Creator2/9
  Bus Selector2/1 -> ratio_AT/1  "<gear_ratio>"
  plant_Connection/14(lock_up_cap) -> Bus Creator2/10
  Bus Selector3/2 -> TransmissionFMU2/2(I_actuator_A1), TMin/2  "<i_actuator>"
  Bus Selector3/1 -> TransmissionFMU2/1(I_EOP_A1), TMin/1  "<i_eop>"
  Bus Creator8/1 -> Bus Selector11/1
  TM Thermal/2(nu_oil_m2ps) -> TransmissionFMU2/4(nu_oil_m2ps), TMin/4  "nu_oil_m2ps"
  TransmissionFMU2/2(Qf_HYD_W) -> TMout/2, Bus Creator3/2
  TransmissionFMU2/3(Qf_SD_PNT_W) -> TMout/3, Bus Creator3/3
  T_PT_TH_K/1(Out1) -> plant_Connection/5(t_engine_water_k)

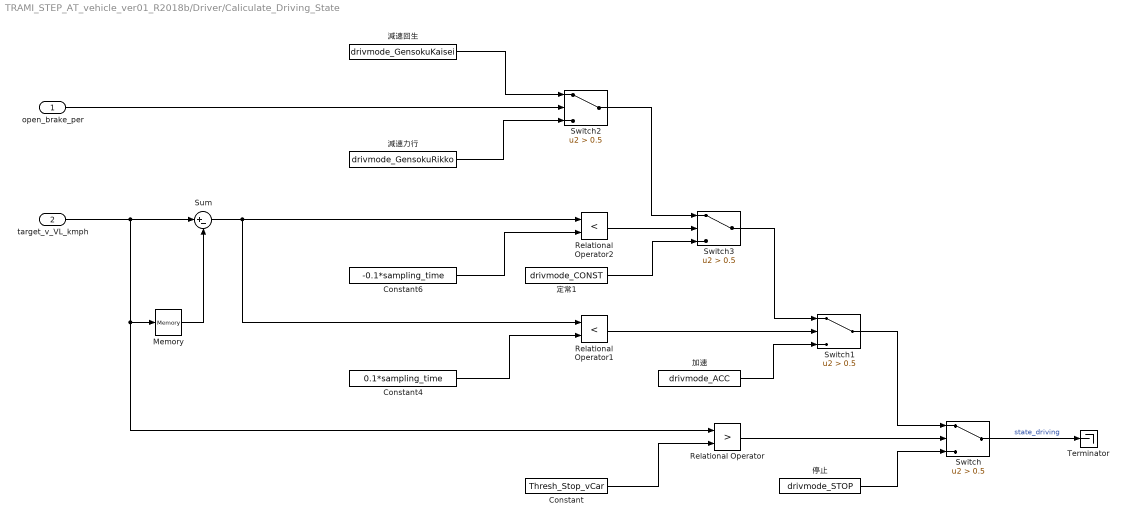
== system TRAMI_STEP_AT_vehicle_ver01_R2018b/Driver/Caliculate_Driving_State ==
  open_brake_per : Inport
  target_v_VL_kmph : Inport  Port=2
  Constant : Constant  Value=Thresh_Stop_vCar
  Constant4 : Constant  Value=0.1*sampling_time
  Constant6 : Constant  Value=-0.1*sampling_time
  Memory : Memory
  Relational Operator : RelationalOperator  Operator=>  OutDataTypeStr=boolean  RndMeth=Nearest
  Relational Operator1 : RelationalOperator  Operator=<  OutDataTypeStr=boolean  RndMeth=Nearest
  Relational Operator2 : RelationalOperator  Operator=<  OutDataTypeStr=boolean  RndMeth=Nearest
  Sum : Sum  Inputs=|+-
  Switch{,1..3} (4 alike) : Switch  Criteria=u2 > Threshold  Threshold=0.5
  Terminator : Terminator
  停止 : Constant  Value=drivmode_STOP
  加速 : Constant  Value=drivmode_ACC
  定常1 : Constant  Value=drivmode_CONST
  減速力行 : Constant  Value=drivmode_GensokuRikko
  減速回生 : Constant  Value=drivmode_GensokuKaisei
  wires:
  Switch/1 -> Terminator/1  "state_driving"
  target_v_VL_kmph/1 -> Relational Operator/1, Memory/1, Sum/1
  Relational Operator1/1 -> Switch1/2
  Constant4/1 -> Relational Operator1/2
  Relational Operator/1 -> Switch/2
  Constant/1 -> Relational Operator/2
  停止/1 -> Switch/3
  Sum/1 -> Relational Operator1/1, Relational Operator2/1
  減速回生/1 -> Switch2/1
  Switch3/1 -> Switch1/1
  Constant6/1 -> Relational Operator2/2
  Memory/1 -> Sum/2
  open_brake_per/1 -> Switch2/2
  減速力行/1 -> Switch2/3
  Relational Operator2/1 -> Switch3/2
  Switch2/1 -> Switch3/1
  定常1/1 -> Switch3/3
  加速/1 -> Switch1/3
  Switch1/1 -> Switch/1

== system TRAMI_STEP_AT_vehicle_ver01_R2018b/Driver/Caliculate_Opeining_Accel ==
  v_VL_PNT_kmph : Inport
  target_v_VL_kmph : Inport  Port=2
  pre_n_eng_rpm : Inport  Port=3
  pre_ratio_DCT : Inport  Port=4
  FB : Subsystem  mask{P_Gain=ACC_P_Gain, D_Gain=ACC_D_Gain, I_Gain=ACC_I_Gain}
      mask prompts: P_Gain "Pゲイン値"; D_Gain "Dゲイン値"; I_Gain "Iゲイン値"
  FF : Subsystem
  Guard_0_100 : Saturate  UpperLimit=ENG_CNT_Throttle_UL  LowerLimit=ENG_CNT_Throttle_LL
  Sum1 : Sum  Inputs=|-+
  Sum3 : Sum  Inputs=++|
  open_accel_per : Outport
  wires:
  Sum1/1 -> FB/1(delta_v_VL_kmph)
  v_VL_PNT_kmph/1 -> FF/1(v_VL_PNT_kmph), Sum1/1
  target_v_VL_kmph/1 -> FF/2(target_v_VL_kmph), Sum1/2
  Sum3/1 -> Guard_0_100/1
  pre_n_eng_rpm/1 -> FF/3(pre_n_eng_rpm)
  pre_ratio_DCT/1 -> FF/4(pre_ratio_DCT)
  FB/1(FB_open_accel_per) -> Sum3/1
  FF/1(FF_open_accel_per) -> Sum3/2
  Guard_0_100/1 -> open_accel_per/1  "open_accel_per"

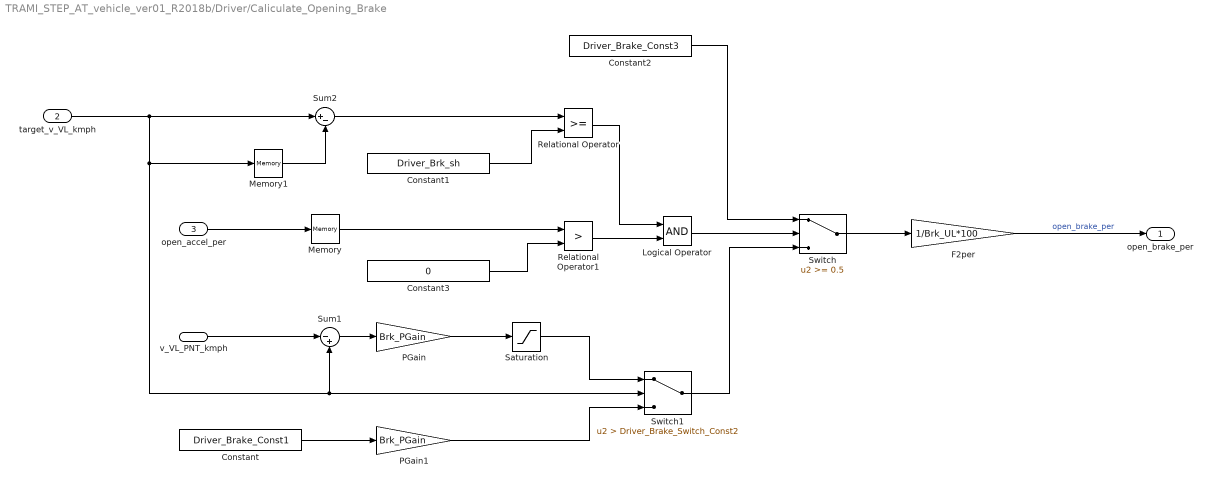
== system TRAMI_STEP_AT_vehicle_ver01_R2018b/Driver/Caliculate_Opening_Brake ==
  v_VL_PNT_kmph : Inport
  target_v_VL_kmph : Inport  Port=2
  open_accel_per : Inport  Port=3
  Constant : Constant  Value=Driver_Brake_Const1
  Constant1 : Constant  Value=Driver_Brk_sh
  Constant2 : Constant  Value=Driver_Brake_Const3
  Constant3 : Constant  Value=0
  F2per : Gain  Gain=1/Brk_UL*100
  Logical Operator : Logic  AllPortsSameDT=off  OutDataTypeStr=boolean
  Memory : Memory
  Memory1 : Memory
  PGain : Gain  Gain=Brk_PGain
  PGain1 : Gain  Gain=Brk_PGain
  Relational Operator : RelationalOperator  OutDataTypeStr=boolean  RndMeth=Nearest
  Relational Operator1 : RelationalOperator  Operator=>  OutDataTypeStr=boolean  RndMeth=Nearest
  Saturation : Saturate  UpperLimit=Brk_UL  LowerLimit=Brk_LL
  Sum1 : Sum  Inputs=|-+
  Sum2 : Sum  Inputs=|+-
  Switch : Switch  Threshold=0.5
  Switch1 : Switch  Criteria=u2 > Threshold  Threshold=Driver_Brake_Switch_Const2
  open_brake_per : Outport
  wires:
  target_v_VL_kmph/1 -> Switch1/2, Sum1/2, Memory1/1, Sum2/1
  Sum1/1 -> PGain/1
  PGain/1 -> Saturation/1
  Constant/1 -> PGain1/1
  PGain1/1 -> Switch1/3
  open_accel_per/1 -> Memory/1
  Memory/1 -> Relational Operator1/1
  Memory1/1 -> Sum2/2
  Switch/1 -> F2per/1
  Sum2/1 -> Relational Operator/1
  Saturation/1 -> Switch1/1
  Switch1/1 -> Switch/3
  Constant2/1 -> Switch/1
  v_VL_PNT_kmph/1 -> Sum1/1
  Constant1/1 -> Relational Operator/2
  Constant3/1 -> Relational Operator1/2
  Relational Operator1/1 -> Logical Operator/2
  Relational Operator/1 -> Logical Operator/1
  Logical Operator/1 -> Switch/2
  F2per/1 -> open_brake_per/1  "open_brake_per"

== system TRAMI_STEP_AT_vehicle_ver01_R2018b/Monitor/Guard_Zero_Devide ==
  note: 0割防止暫定処置
  In1 : Inport
  In2 : Inport  Port=2
  Constant1 : Constant  Value=fuel_0guard
  Constant2 : Constant  Value=fuelcomsnp_0
  Divide : Product  Inputs=*/
  MinMax : MinMax  Function=max  Inputs=2
  Relational Operator : RelationalOperator  OutDataTypeStr=boolean  RndMeth=Nearest
  Switch1 : Switch  Criteria=u2 > Threshold  Threshold=0.5
  Out1 : Outport
  wires:
  In2/1 -> MinMax/1, Relational Operator/1
  In1/1 -> Divide/1
  Switch1/1 -> Out1/1  "燃費[km/l]"
  Divide/1 -> Switch1/1  "燃費[km/l]"
  Constant2/1 -> Switch1/3
  Relational Operator/1 -> Switch1/2
  MinMax/1 -> Divide/2
  Constant1/1 -> MinMax/2, Relational Operator/2

== system TRAMI_STEP_AT_vehicle_ver01_R2018b/Vehicle/ALT_CNT ==
  note: 【発電禁止条件】
      | 下記条件いずれかが成立時はオルタネータの発電を禁止する
      |   (2)エンジン停止中
      |   (3)エンジン始動中(下記エンジン回転数で判定)
      |      ene ≦ ALT_ON_RPM_HYS(1000[rpm])
      |                    ヒスあり(400[rpm])
  note: 【強制回生モード切替条件】
  note: 【回生モード切替条件】
      | 減速時FC中
  note: 例) 12[V]
  note: 例) 14[V]
  note: 例) 13.5[V]
  flag_fuelcut : Inport
  flag_IdleStop : Inport  Port=2
  n_eng_rpm : Inport  Port=3
  SOC_BT_PNT_Lo_PCT : Inport  Port=4
  Constant : Constant  Value=ALT_CNT_Alter_V_Kaisei_V
  Constant1 : Constant  Value=ALT_CNT_V_Battely_Kudo_V
  Constant2 : Constant  Value=ALT_CNT_flag_disable_kaisei
  Constant3 : Constant  Value=ALT_CNT_Alter_V_BASE_V
  Constant4 : Constant  Value=BT_PNT_Lo_SOC_MAX_lo_batt
  Logical Operator : Logic  Operator=OR  Inputs=3  AllPortsSameDT=off  OutDataTypeStr=boolean
  Logical Operator1 : Logic  AllPortsSameDT=off  OutDataTypeStr=boolean
  Logical Operator2 : Logic  Operator=NOT  AllPortsSameDT=off  OutDataTypeStr=boolean
  Relational Operator : RelationalOperator  OutDataTypeStr=boolean  RndMeth=Nearest
  Relay1 : Relay  OnSwitchValue=ALT_CNT_ALT_ON_RPM_HYS_rpm  OffSwitchValue=ALT_CNT_ALT_OFF_RPM_HYS_rpm  OnOutputValue=0  OffOutputValue=1
  Switch1 : Switch  Criteria=u2 > Threshold  Threshold=0.5
  Switch3 : Switch  Criteria=u2 > Threshold  Threshold=0.5
  target_volt_ALT_V : Outport
  wires:
  Constant1/1 -> Switch1/3
  Switch3/1 -> target_volt_ALT_V/1  "target_volt_ALT_V"
  Constant4/1 -> Relational Operator/2
  flag_IdleStop/1 -> Logical Operator/1
  Relay1/1 -> Logical Operator/2
  Relational Operator/1 -> Logical Operator/3
  Constant/1 -> Switch1/1
  flag_fuelcut/1 -> Logical Operator1/1
  Logical Operator/1 -> Logical Operator2/1
  Constant3/1 -> Switch3/1
  Constant2/1 -> Switch3/2
  Switch1/1 -> Switch3/3
  Logical Operator1/1 -> Switch1/2
  Logical Operator2/1 -> Logical Operator1/2
  n_eng_rpm/1 -> Relay1/1
  SOC_BT_PNT_Lo_PCT/1 -> Relational Operator/1

== system TRAMI_STEP_AT_vehicle_ver01_R2018b/Vehicle/ALT_PNT ==
  note: 発電する為のトルクが負
  note: スルー量が出力の場合、発電する方向が正
  target_volt_ALT_V : Inport
  w_ENG_PNT_radps : Inport  Port=2
  volt_BT_PNT_Lo_V : Inport  Port=3
  Gain : Gain  Gain=-1
  Memory1 : Memory
  P_cal : METI_Lib_vehicle_model/P_cal  Type_energy=回転運動  Type_output_energy=出力  Power_name=Po_  t_Workspace_Name=ALT_PNT_MECK  P_VariableName=Po_ALT_PNT_MECK  Across_VariableName=w_ALT_PNT_MECK  Throgh_VariableName=tq_ALT_PNT_MECK
      settings: SourceProductName=The database C:\Users\k-uekata\AppData\Roaming\MathWorks\MATLAB\R2018b\slblocks_master.db is locked, or a table in the database is locked. (database is locked)
  P_cal1 : METI_Lib_vehicle_model/P_cal  Type_energy=電気  Type_output_energy=出力  Power_name=Po_  t_Workspace_Name=ALT_PNT_ELEC  P_VariableName=Po_ALT_PNT_ELEC  Across_VariableName=V_ALT_PNT_ELEC  Throgh_VariableName=I_ALT_PNT_ELEC
      settings: SourceProductName=The database C:\Users\k-uekata\AppData\Roaming\MathWorks\MATLAB\R2018b\slblocks_master.db is locked, or a table in the database is locked. (database is locked)
  Subsystem : Subsystem
  Terminator : Terminator
  Terminator1 : Terminator
  pulley_slave : Subsystem
  trq_ALT_PNT_Nm : Outport
  current_ALT_PNT_A : Outport  Port=2
  tag scope: tScope_V_ALT=global
  wires:
  Memory1/1 -> Subsystem/2(w_ROT_slavepulley12)
  Subsystem/1(current_ALT_PNT_A) -> P_cal1/2, current_ALT_PNT_A/1
  Gain/1 -> trq_ALT_PNT_Nm/1  "trq_ALT_PNT_Nm"
  pulley_slave/1(trq_slavepulley11) -> Gain/1
  w_ENG_PNT_radps/1 -> pulley_slave/1(w_ENG_PNT_radps)
  Subsystem/2(trq_trqsource) -> P_cal/2, pulley_slave/2(trq_slavepulley12)
  volt_BT_PNT_Lo_V/1 -> [tScope_V_ALT], P_cal1/1, Subsystem/3(volt_BT_PNT_Lo_V)
  P_cal1/1 -> Terminator1/1
  P_cal/1 -> Terminator/1
  pulley_slave/2(w_slavepulley12) -> P_cal/1, Memory1/1
  target_volt_ALT_V/1 -> Subsystem/1(target_volt_ALT_V)

== system TRAMI_STEP_AT_vehicle_ver01_R2018b/Vehicle/BK_CNT ==
  open_brake_per_in : Inport
  open_brake_per : Outport
  wires:
  open_brake_per_in/1 -> open_brake_per/1

== system TRAMI_STEP_AT_vehicle_ver01_R2018b/Vehicle/BK_PNT ==
  note: 制動力
  open_brake_per : Inport
  w_TR_PNT_radps : Inport  Port=2
  Constant2 : Constant  Value=tire_r
  Gain : Gain  Gain=-1
  Product6 : Product  RndMeth=Zero
  Q_cal3 : METI_Lib_vehicle_model/P_cal  Type_energy=回転運動  Type_output_energy=損失  Power_name=Pl_  t_Workspace_Name=BK_PNT_MECK_LOSS  P_VariableName=Pl_BK_PNT_MECK_LOSS  Across_VariableName=w_BK_PNT_MECK_LOSS  Throgh_VariableName=tq_BK_PNT_MECK_LOSS
      settings: SourceProductName=The database C:\Users\k-uekata\AppData\Roaming\MathWorks\MATLAB\R2018b\slblocks_master.db is locked, or a table in the database is locked. (database is locked)
  Terminator1 : Terminator
  Transfer Fcn : TransferFcn  Denominator=[BK_PNT_Tau_brake 1]
  per2F : Gain  Gain=BK_PNT_Pow_UL/100
  trq_BK_PNT_Nm : Outport
  wires:
  Q_cal3/1 -> Terminator1/1
  Transfer Fcn/1 -> Product6/2
  Constant2/1 -> Product6/1
  Product6/1 -> Gain/1, Q_cal3/2
  w_TR_PNT_radps/1 -> Q_cal3/1
  open_brake_per/1 -> per2F/1
  Gain/1 -> trq_BK_PNT_Nm/1  "trq_BK_PNT_Nm"
  per2F/1 -> Transfer Fcn/1

== system TRAMI_STEP_AT_vehicle_ver01_R2018b/Vehicle/BT_PNT_Lo ==
  note: SOC算出
  note: 内部抵抗
  note: OCV電圧算出
  Current_Chg_Lo_BT_A : Inport
  Cal_SOC : Subsystem
  Capa_batt(Ah) : Constant  Value=BT_PNT_Lo_Capa_lo_batt_F
  Memory6 : Memory  InitialCondition=BT_PNT_Lo_V_start_ocv  InheritSampleTime=on
  P_cal : METI_Lib_vehicle_model/P_cal  Type_energy=電気  Type_output_energy=出力  Power_name=Po_  t_Workspace_Name=BT_PNT_Lo_ELEC  P_VariableName=Po_BT_PNT_Lo_ELEC  Across_VariableName=V_BT_PNT_Lo_ELEC  Throgh_VariableName=I_BT_PNT_Lo_ELEC
      settings: SourceProductName=The database C:\Users\k-uekata\AppData\Roaming\MathWorks\MATLAB\R2018b\slblocks_master.db is locked, or a table in the database is locked. (database is locked)
  P_cal1 : METI_Lib_vehicle_model/P_cal  Type_energy=電気  Type_output_energy=損失  Power_name=Pl_  t_Workspace_Name=BT_PNT_Lo_ELEC_LOSS  P_VariableName=Pl_BT_PNT_Lo_ELEC_LOSS  Across_VariableName=V_BT_PNT_Lo_ELEC_LOSS  Throgh_VariableName=I_BT_PNT_Lo_ELEC_LOSS
      settings: SourceProductName=The database C:\Users\k-uekata\AppData\Roaming\MathWorks\MATLAB\R2018b\slblocks_master.db is locked, or a table in the database is locked. (database is locked)
  SOC_MAX(%) : Constant  Value=BT_PNT_Lo_SOC_MAX_lo_batt
  SOC_MIN(%) : Constant  Value=BT_PNT_Lo_SOC_MIN_lo_batt
  SOC_START(%) : Constant  Value=BT_PNT_Lo_SOC_START_lo_batt
  Subsystem : Subsystem
  Sum : Sum  Inputs=|++
  Terminator1 : Terminator
  Terminator2 : Terminator
  map_OCV : Lookup  InputValues=BT_PNT_Lo_ocv_SOC_lo_batt_OCV_V_table_x_SOC  Table=BT_PNT_Lo_ocv_SOC_lo_batt_OCV_V_table  LookUpMeth=Interpolation-Use End Values
  volt_BT_PNT_Lo_V : Outport
  SOC_BT_PNT_Lo_PCT : Outport  Port=2
  tag scope: tScope_SOC_Batt=global
  wires:
  Sum/1 -> Memory6/1
  Capa_batt(Ah)/1 -> Cal_SOC/2(Capa_batt)
  SOC_START(%)/1 -> Cal_SOC/3(SOC_st)
  SOC_MAX(%)/1 -> Cal_SOC/4(SOC_MAX)
  SOC_MIN(%)/1 -> Cal_SOC/5(SOC_MIN)
  Memory6/1 -> volt_BT_PNT_Lo_V/1, P_cal/1  "volt_BT_PNT_Lo_V"
  map_OCV/1 -> Sum/1
  Subsystem/1(V_BT_PNT_Lo_V) -> P_cal1/1, Sum/2
  P_cal/1 -> Terminator2/1
  P_cal1/1 -> Terminator1/1
  Current_Chg_Lo_BT_A/1 -> P_cal/2, P_cal1/2, Subsystem/1(I_BT_PNT_Lo_A), Cal_SOC/1(I_Lo_BT_PNT_A)
  Cal_SOC/1(SOC_out) -> SOC_BT_PNT_Lo_PCT/1, map_OCV/1, [tScope_SOC_Batt]  "SOC_BT_PNT_Lo_PCT"

== system TRAMI_STEP_AT_vehicle_ver01_R2018b/Vehicle/EL_PNT ==
  note: 低圧側電気負荷
  volt_BT_PNT_Lo_V : Inport
  Add : Sum  Inputs=+-|
  Ground : Ground
  P_cal1 : METI_Lib_vehicle_model/P_cal  Type_energy=電気  Type_output_energy=損失  Power_name=Pl_  t_Workspace_Name=EL_PNT_ELEC_LOSS  P_VariableName=Pl_EL_PNT_ELEC_LOSS  Across_VariableName=V_EL_PNT_ELEC_LOSS  Throgh_VariableName=I_EL_PNT_ELEC_LOSS
      settings: SourceProductName=The database C:\Users\k-uekata\AppData\Roaming\MathWorks\MATLAB\R2018b\slblocks_master.db is locked, or a table in the database is locked. (database is locked)
  Product3 : Product  Inputs=*/  RndMeth=Zero
  Resistance2 : Constant  Value=EL_PNT_R_bodyelec_lo_ohm
  Terminator1 : Terminator
  current_EL_PNT_A : Outport
  wires:
  Product3/1 -> P_cal1/2, current_EL_PNT_A/1  "current_EL_PNT_A"
  volt_BT_PNT_Lo_V/1 -> Add/1
  Ground/1 -> Add/2
  Add/1 -> P_cal1/1, Product3/1
  Resistance2/1 -> Product3/2
  P_cal1/1 -> Terminator1/1

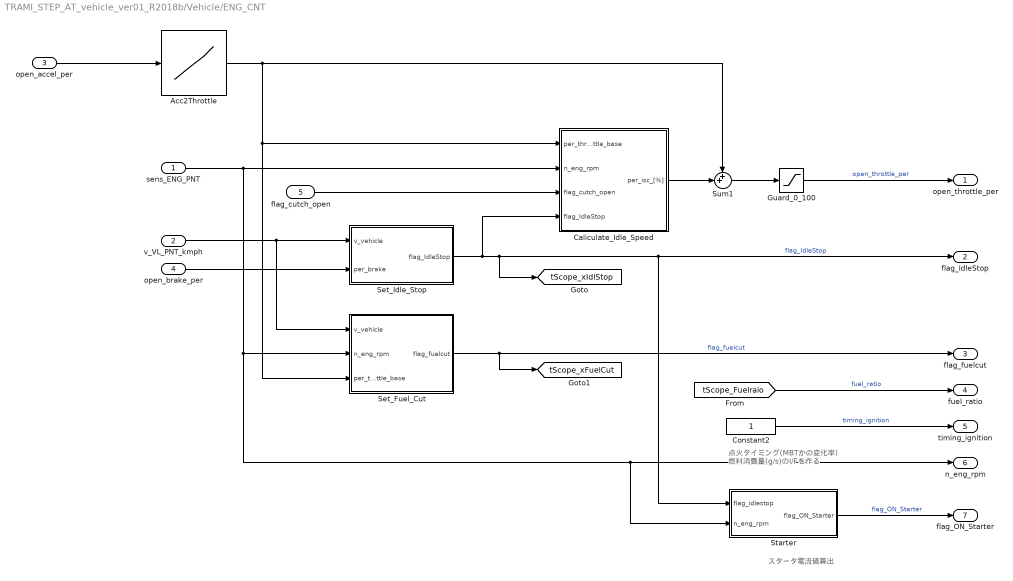
== system TRAMI_STEP_AT_vehicle_ver01_R2018b/Vehicle/ENG_CNT ==
  note: 点火タイミング(MBTかの変化率)
      | 燃料消費量(g/s)のI/Fを作る
  note: スタータ電流値算出
  sens_ENG_PNT : Inport
  v_VL_PNT_kmph : Inport  Port=2
  open_accel_per : Inport  Port=3
  open_brake_per : Inport  Port=4
  flag_cutch_open : Inport  Port=5
  Acc2Throttle : Lookup_n-D  NumberOfTableDimensions=1  BreakpointsForDimension1=[ENG_CNT_Accel_LL:ENG_CNT_Accel_UL]  Table=[ENG_CNT_Throttle_LL:ENG_CNT_Throttle_UL]  RndMeth=Simplest  InputSameDT=on
  Caliculate_Idle_Speed : Subsystem
  Constant2 : Constant
  Guard_0_100 : Saturate  UpperLimit=ENG_CNT_Throttle_UL  LowerLimit=ENG_CNT_Throttle_LL
  Set_Fuel_Cut : Subsystem
  Set_Idle_Stop : Subsystem
  Starter : Subsystem
  Sum1 : Sum  Inputs=++|
  open_throttle_per : Outport
  flag_IdleStop : Outport  Port=2
  flag_fuelcut : Outport  Port=3
  fuel_ratio : Outport  Port=4
  timing_ignition : Outport  Port=5
  n_eng_rpm : Outport  Port=6
  flag_ON_Starter : Outport  Port=7
  tag scope: tScope_xFuelCut=global, tScope_xIdlStop=global
  wires:
  Set_Idle_Stop/1(flag_IdleStop) -> Caliculate_Idle_Speed/4(flag_IdleStop), flag_IdleStop/1, Starter/1(flag_idlestop), [tScope_xIdlStop]  "flag_IdleStop"
  Caliculate_Idle_Speed/1(per_isc_[%]) -> Sum1/2
  Sum1/1 -> Guard_0_100/1
  Acc2Throttle/1 -> Sum1/1, Caliculate_Idle_Speed/1(per_throttle_base), Set_Fuel_Cut/3(per_throttle_base)
  [tScope_Fuelraio] -> fuel_ratio/1  "fuel_ratio"
  Constant2/1 -> timing_ignition/1  "timing_ignition"
  Set_Fuel_Cut/1(flag_fuelcut) -> flag_fuelcut/1, [tScope_xFuelCut]  "flag_fuelcut"
  Guard_0_100/1 -> open_throttle_per/1  "open_throttle_per"
  sens_ENG_PNT/1 -> Caliculate_Idle_Speed/2(n_eng_rpm), Set_Fuel_Cut/2(n_eng_rpm), n_eng_rpm/1, Starter/2(n_eng_rpm)
  open_brake_per/1 -> Set_Idle_Stop/2(per_brake)
  open_accel_per/1 -> Acc2Throttle/1
  v_VL_PNT_kmph/1 -> Set_Idle_Stop/1(v_vehicle), Set_Fuel_Cut/1(v_vehicle)
  Starter/1(flag_ON_Starter) -> flag_ON_Starter/1  "flag_ON_Starter"
  flag_cutch_open/1 -> Caliculate_Idle_Speed/3(flag_cutch_open)

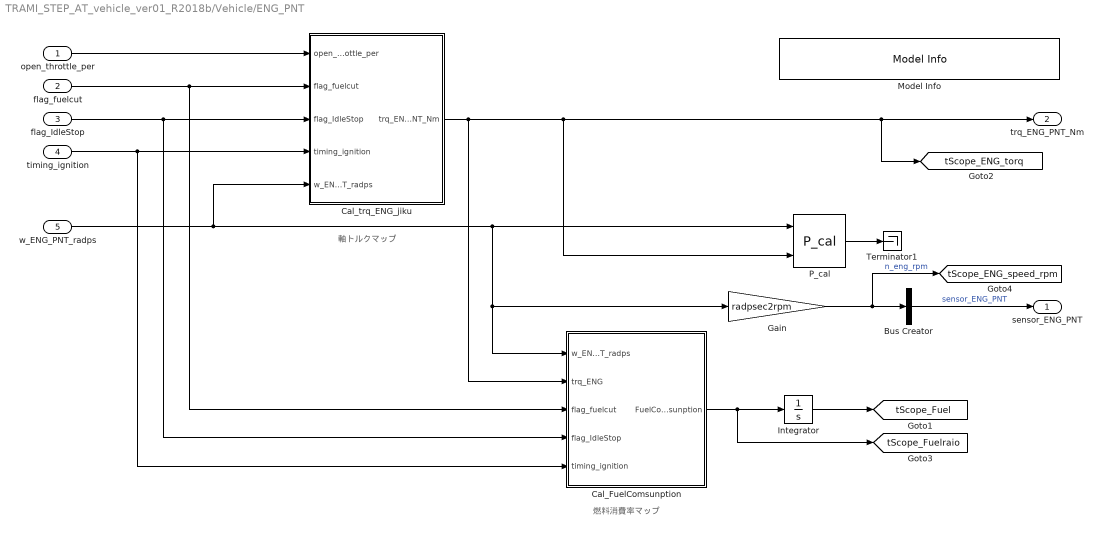
== system TRAMI_STEP_AT_vehicle_ver01_R2018b/Vehicle/ENG_PNT ==
  note: 軸トルクマップ
  note: 燃料消費率マップ
  open_throttle_per : Inport
  flag_fuelcut : Inport  Port=2
  flag_IdleStop : Inport  Port=3
  timing_ignition : Inport  Port=4
  w_ENG_PNT_radps : Inport  Port=5
  Bus Creator : BusCreator  Inputs=1
  Cal_FuelComsunption : Subsystem
  Cal_trq_ENG_jiku : Subsystem
  Gain : Gain  Gain=radpsec2rpm
  Integrator : Integrator
  Model Info : simulink/Model-Wide Utilities/Model Info  Frame=on  DisplayStringWithTags=【注記】 ・エンジンモデルはトルク出力動作させる側が正  HorizontalTextAlignment=Left  LeftAlignmentValue=0.02
  P_cal : METI_Lib_vehicle_model/P_cal  Type_energy=回転運動  Type_output_energy=出力  Power_name=Po_  t_Workspace_Name=ENG_PNT_MECK  P_VariableName=Po_ENG_PNT_MECK  Across_VariableName=w_ENG_PNT_MECK  Throgh_VariableName=tq_ENG_PNT_MECK
      settings: SourceProductName=The database C:\Users\k-uekata\AppData\Roaming\MathWorks\MATLAB\R2018b\slblocks_master.db is locked, or a table in the database is locked. (database is locked)
  Terminator1 : Terminator
  sensor_ENG_PNT : Outport
  trq_ENG_PNT_Nm : Outport  Port=2
  tag scope: tScope_ENG_speed_rpm=global, tScope_ENG_torq=global, tScope_Fuel=global, tScope_Fuelraio=global
  wires:
  Cal_FuelComsunption/1(FuelComsunption) -> [tScope_Fuelraio], Integrator/1
  Integrator/1 -> [tScope_Fuel]
  w_ENG_PNT_radps/1 -> Cal_trq_ENG_jiku/5(w_ENG_PNT_radps), P_cal/1, Gain/1, Cal_FuelComsunption/1(w_ENG_PNT_radps)
  P_cal/1 -> Terminator1/1
  flag_fuelcut/1 -> Cal_trq_ENG_jiku/2(flag_fuelcut), Cal_FuelComsunption/3(flag_fuelcut)
  flag_IdleStop/1 -> Cal_FuelComsunption/4(flag_IdleStop), Cal_trq_ENG_jiku/3(flag_IdleStop)
  open_throttle_per/1 -> Cal_trq_ENG_jiku/1(open_throttle_per)
  Cal_trq_ENG_jiku/1(trq_ENG_PNT_Nm) -> Cal_FuelComsunption/2(trq_ENG), P_cal/2, [tScope_ENG_torq], trq_ENG_PNT_Nm/1
  timing_ignition/1 -> Cal_FuelComsunption/5(timing_ignition), Cal_trq_ENG_jiku/4(timing_ignition)
  Gain/1 -> [tScope_ENG_speed_rpm], Bus Creator/1  "n_eng_rpm"
  Bus Creator/1 -> sensor_ENG_PNT/1  "sensor_ENG_PNT"

== system TRAMI_STEP_AT_vehicle_ver01_R2018b/Vehicle/ST_PNT ==
  flag_ON_Starter : Inport
  w_ENG_PNT_radps : Inport  Port=2
  volt_BT_PNT_Lo_V : Inport  Port=3
  Constant1 : Constant  Value=OFF
  Constant6 : Constant  Value=OFF
  Gain : Gain  Gain=1/ST_PNT_Starter_Res_ohm
  Switch : Switch  Criteria=u2 > Threshold  Threshold=0.5
  Terminator : Terminator
  trq__ST_PNT_Nm : Outport
  current_ST_PNT_A : Outport  Port=2
  wires:
  volt_BT_PNT_Lo_V/1 -> Switch/1
  Switch/1 -> Gain/1
  Gain/1 -> current_ST_PNT_A/1  "current_ST_PNT_A"
  Constant6/1 -> Switch/3
  flag_ON_Starter/1 -> Switch/2
  Constant1/1 -> trq__ST_PNT_Nm/1  "trq__ST_PNT_Nm"
  w_ENG_PNT_radps/1 -> Terminator/1

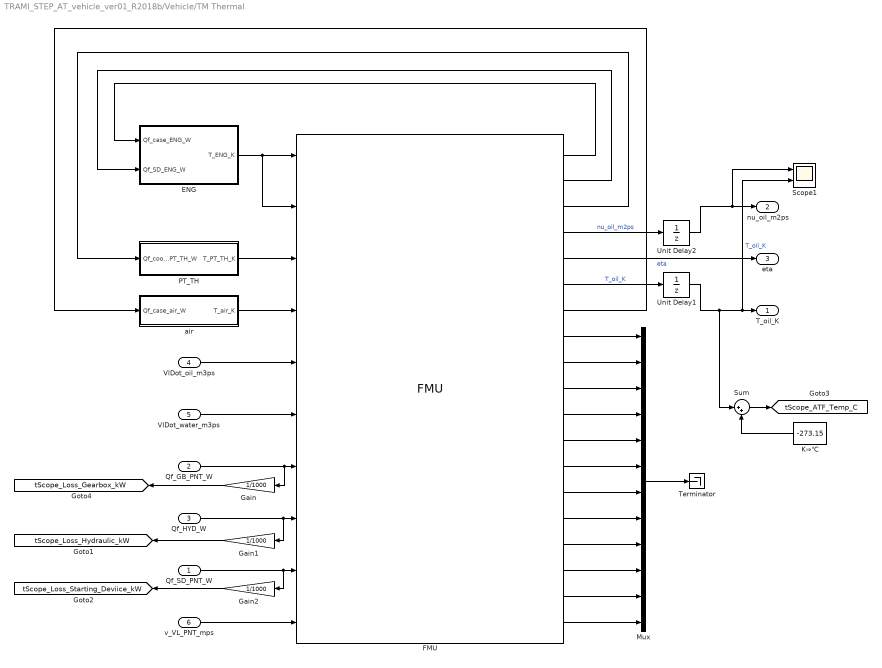
== system TRAMI_STEP_AT_vehicle_ver01_R2018b/Vehicle/TM Thermal ==
  Qf_SD_PNT_W : Inport
      settings: AttributesFormatString=|
      | %<Tag>
      | Priority=<%<Priority>>
  Qf_GB_PNT_W : Inport  Port=2
      settings: AttributesFormatString=|
      | %<Tag>
      | Priority=<%<Priority>>
  Qf_HYD_W : Inport  Port=3
      settings: AttributesFormatString=|
      | %<Tag>
      | Priority=<%<Priority>>
  VlDot_oil_m3ps : Inport  Port=4
      settings: AttributesFormatString=|
      | %<Tag>
      | Priority=<%<Priority>>
  VlDot_water_m3ps : Inport  Port=5
      settings: AttributesFormatString=|
      | %<Tag>
      | Priority=<%<Priority>>
  v_VL_PNT_mps : Inport  Port=6
      settings: AttributesFormatString=|
      | %<Tag>
      | Priority=<%<Priority>>
  ENG : Subsystem
  FMU : FMU  FMUName=ThermalModelAll_CS.fmu  FMUDebugLogging=on  FMUMode=CoSimulation  c1=5000  T0=300  R1=100  T1=300  R2=0.10  R3=100  R4=100  R5=0.006  table1_1_1__1_1_=0.  table1_1_2__1_2_=0.022  table1_2_1__2_1_=10.  table1_2_2__2_2_=0.021  table1_3_1__3_1_=20.  table1_3_2__3_2_=0.021  table1_4_1__4_1_=30.  table1_4_2__4_2_=0.020  table1_5_1__5_1_=40.  table1_5_2__5_2_=0.019  table1_6_1__6_1_=50.  table1_6_2__6_2_=0.018  table1_7_1__7_1_=60.  table1_7_2__7_2_=0.017  table1_8_1__8_1_=70.  table1_8_2__8_2_=0.016  table1_9_1__9_1_=80.  table1_9_2__9_2_=0.015  table1_10_1__10_1_=90.  table1_10_2__10_2_=0.014  table1_11_1__11_1_=100.  table1_11_2__11_2_=0.013  table1_12_1__12_1_=110.  table1_12_2__12_2_=0.012  table1_13_1__13_1_=120.  table1_13_2__13_2_=0.012  table1_14_1__14_1_=130.  table1_14_2__14_2_=0.011  table1_15_1__15_1_=140.  table1_15_2__15_2_=0.011  table1_16_1__16_1_=150.  table1_16_2__16_2_=0.010  table1_17_1__17_1_=160.  table1_17_2__17_2_=0.010  c3=15000  T2=300  fileName1=./DATA/thResistanceOilColler1.txt  tableName1=thResistanceOilColler1  T3=300  c4=10000  R6=0.0007  R7=0.05  Nutable1_1_1__1_1_=-30.  Nutable1_1_2__1_2_=70  Nutable1_2_1__2_1_=0.  Nutable1_2_2__2_2_=70  Nutable1_3_1__3_1_=20.  Nutable1_3_2__3_2_=70  Nutable1_4_1__4_1_=40.  Nutable1_4_2__4_2_=40  Nutable1_5_1__5_1_=60.  Nutable1_5_2__5_2_=23  Nutable1_6_1__6_1_=80.  Nutable1_6_2__6_2_=13  Nutable1_7_1__7_1_=100.  Nutable1_7_2__7_2_=7.5  Nutable1_8_1__8_1_=120.  Nutable1_8_2__8_2_=7.5  EtaTable1_1_1__1_1_=-30.  EtaTable1_1_2__1_2_=70  EtaTable1_2_1__2_1_=0.  EtaTable1_2_2__2_2_=70  EtaTable1_3_1__3_1_=20.  EtaTable1_3_2__3_2_=70  EtaTable1_4_1__4_1_=40.  EtaTable1_4_2__4_2_=40  EtaTable1_5_1__5_1_=60.  EtaTable1_5_2__5_2_=23  EtaTable1_6_1__6_1_=80.  EtaTable1_6_2__6_2_=13  EtaTable1_7_1__7_1_=100.  EtaTable1_7_2__7_2_=7.5  EtaTable1_8_1__8_1_=120.  EtaTable1_8_2__8_2_=7.5  kDammy=1.  c2=30000  settings_dtMin=1e-08  settings_dtMax=0.01  settings_absTol=1e-05  settings_relTol=1e-05  settings_iMode=int32(1)  settings_maxOrder=int32(5)  mask(ThermalModelAll [Co-Simulation, v2.0]){}
      mask Display: disp('ThermalModelAll');
  Gain : Gain  Gain=1/1000
  Gain1 : Gain  Gain=1/1000
  Gain2 : Gain  Gain=1/1000
  K⇒℃ : Constant  Value=-273.15
  Mux : Mux  Inputs=12
  PT_TH : Subsystem
  Scope1 : Scope  NumInputPorts=2
  Sum : Sum  Inputs=|++
  Terminator : Terminator
  Unit Delay1 : UnitDelay  InitialCondition=8e-5  SampleTime=-1
  Unit Delay2 : UnitDelay  InitialCondition=8e-5  SampleTime=-1
  air : Subsystem
  T_oil_K : Outport
      settings: AttributesFormatString=|
      | %<Tag>
      | Priority=<%<Priority>>
  nu_oil_m2ps : Outport  Port=2
      settings: AttributesFormatString=|
      | %<Tag>
      | Priority=<%<Priority>>
  eta : Outport  Port=3
      settings: AttributesFormatString=|
      | %<Tag>
      | Priority=<%<Priority>>
  tag scope: tScope_ATF_Temp_C=global, tScope_Loss_Gearbox_kW=global, tScope_Loss_Hydraulic_kW=global, tScope_Loss_Starting_Deviice_kW=global
  wires:
  ENG/1(T_ENG_K) -> FMU/2, FMU/1
  PT_TH/1(T_PT_TH_K) -> FMU/3
  v_VL_PNT_mps/1 -> FMU/10
  Qf_SD_PNT_W/1 -> Gain2/1, FMU/9
  VlDot_oil_m3ps/1 -> FMU/5
  VlDot_water_m3ps/1 -> FMU/6
  Qf_HYD_W/1 -> Gain1/1, FMU/8
  air/1(T_air_K) -> FMU/4
  FMU/5 -> eta/1  "eta"
  FMU/4 -> Unit Delay2/1  "nu_oil_m2ps"
  FMU/1 -> ENG/1(Qf_case_ENG_W)
  FMU/2 -> ENG/2(Qf_SD_ENG_W)
  FMU/3 -> PT_TH/1(Qf_cooler_PT_TH_W)
  FMU/7 -> air/1(Qf_case_air_W)
  FMU/8 -> Mux/1
  FMU/9 -> Mux/2
  FMU/10 -> Mux/3
  FMU/12 -> Mux/5
  FMU/11 -> Mux/4
  FMU/13 -> Mux/6
  FMU/14 -> Mux/7
  FMU/15 -> Mux/8
  FMU/16 -> Mux/9
  FMU/17 -> Mux/10
  FMU/18 -> Mux/11
  FMU/19 -> Mux/12
  Mux/1 -> Terminator/1
  FMU/6 -> Unit Delay1/1  "T_oil_K"
  Qf_GB_PNT_W/1 -> Gain/1, FMU/7
  Unit Delay1/1 -> Sum/1, Scope1/2, T_oil_K/1  "T_oil_K"
  Unit Delay2/1 -> Scope1/1, nu_oil_m2ps/1
  Gain/1 -> [tScope_Loss_Gearbox_kW]
  Gain1/1 -> [tScope_Loss_Hydraulic_kW]
  Gain2/1 -> [tScope_Loss_Starting_Deviice_kW]
  Sum/1 -> [tScope_ATF_Temp_C]
  K⇒℃/1 -> Sum/2
